simulink model "extract_state"  (R2017a)
settings: Solver=VariableStepAuto  StartTime=0.0  StopTime=10.0  RelTol=1e-3
settings Model: Creator=User  LastModifiedBy=User

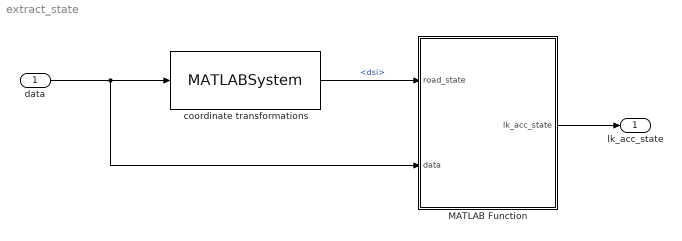
== system extract_state ==
  data : Inport  OutDataTypeStr=Bus: DataBus
  MATLAB Function : MATLAB Function  TreatAsAtomicUnit=on
  coordinate transformations : MATLABSystem  System=road  lat0=42.30095833  long0=-83.69758056  h0=0  pathfile=C:/MKZ/mcity/fixed_path.ascii  N_path=3  N_interp=10  dt=0.1  SimulateUsing=Code generation
      mask Type: road
      mask Display:
      | disp('road');
      | port_label('input',1,'data');
      | port_label('output',1,'road_state');
  lk_acc_state : Outport  OutDataTypeStr=Bus: LKACCBus
  wires:
  coordinate transformations/1 -> MATLAB Function/1(road_state)  "<dsi>"
  data/1 -> coordinate transformations/1, MATLAB Function/2(data)
  MATLAB Function/1(lk_acc_state) -> lk_acc_state/1

== matlab function extract_state/MATLAB Function ==
  data: road_state input Bus: RoadBus; data input Bus: DataBus; lk_acc_state output Bus: LKACCBus
function lk_acc_state  = get_states(road_state, data)
    
    % unit vector direction of road
    road_unit = [road_state.d_road_x; road_state.d_road_y]/...
                norm([road_state.d_road_x; road_state.d_road_y]);

    % relative position
    rel_pos = [road_state.car_x - road_state.road_x;
               road_state.car_y - road_state.road_y];
    
    % velocity in global frame
    global_vel = [data.Vx*cos(data.Yaw)-data.Vy*sin(data.Yaw);
                  data.Vx*sin(data.Yaw)+data.Vy*cos(data.Yaw)];
    
    % yaw angles
    normDeg = @(x) pi-mod(pi-x, 2*pi);
    
    road_yaw = cart2pol(road_unit(1), road_unit(2));
    global_yaw = normDeg(normDeg(data.Yaw) + cart2pol(data.Vx, data.Vy));
    
    dPsi = normDeg(global_yaw - road_yaw);
    
    % assign
    lk_acc_state.y = det([road_unit rel_pos]);
    lk_acc_state.dy = det([road_unit global_vel]);
    lk_acc_state.mu = data.Vx;
    lk_acc_state.nu = data.Vy;
    lk_acc_state.dPsi = dPsi;
    lk_acc_state.r = data.YawRate;
    lk_acc_state.h = 8;
    lk_acc_state.r_d = road_state.kappa * norm(global_vel);
